simulink model "MainSim"  (R2024a)
settings: Solver=ode4  StartTime=0.0  StopTime=simtime  FixedStep=0.1  RelTol=1e-3
values from neighbouring files (symbols this model uses):
  C = [1 0 0 0 0 0 -1 0 0 0 0 0 ... (45 elements, 5x9)]    [C.mat]
undefined symbols (not defined in the file or in its folder): Ki, Kp, ssest, syys, utrim, xtrim
libraries: neural x680
(part 1 of 12)
settings Model: Creator=soeta  LastModifiedBy=soeta
settings DataIOCC: ReturnWorkspaceOutputs=off

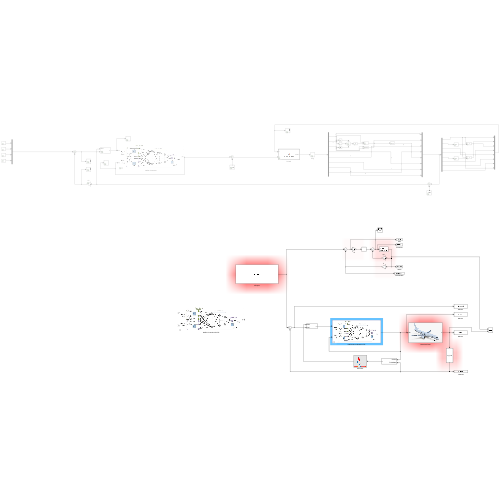
[thumbnail: Simulink's stored preview of the top-level diagram]
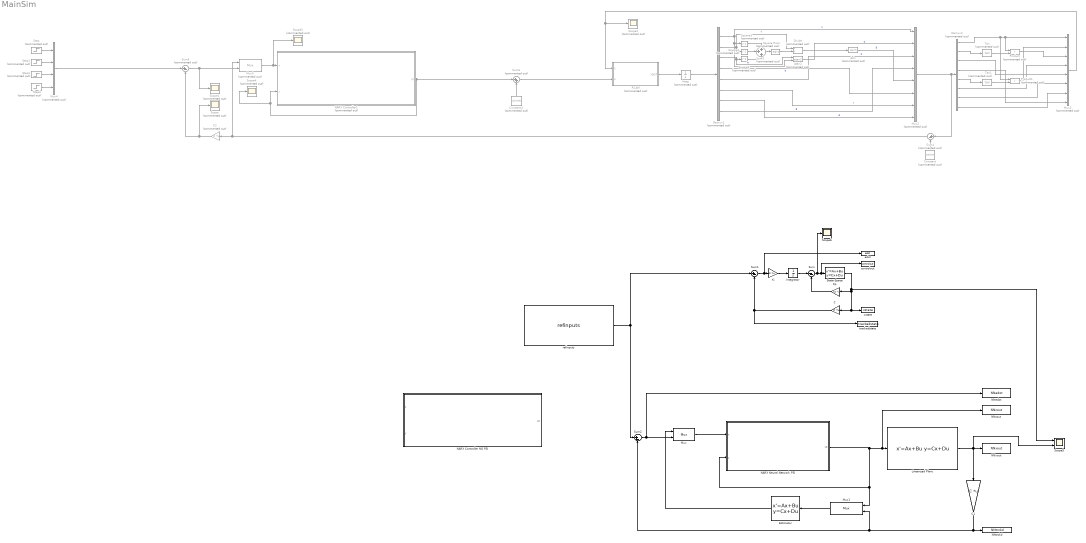
== system MainSim ==
  Asin : Trigonometry  Commented=on  Operator=asin
  Atan2 : Trigonometry  Commented=on  Operator=atan2
  C : Gain  Gain=C  Multiplication=Matrix(K*u)
  C1 : Gain  Gain=C  Multiplication=Matrix(K*u)
      mask Display: fprintf('u γ β Φ')
  C2 : Gain  Commented=on  Gain=C  Multiplication=Matrix(K*u)
  Constant : Constant  Commented=on  Value=xtrim
  Constant1 : Constant  Commented=on  Value=utrim
  Demux1 : Demux  Commented=on  Outputs=8
  Demux2 : Demux  Commented=on  Outputs=8
  Divide : Product  Commented=on  Inputs=*/
  Estimator : StateSpace  A=ssest.A  B=ssest.B  C=ssest.C  D=ssest.D  InitialCondition=0
      mask Display: image('icon_Est.png');
  Integ : Integrator  Commented=on  InitialCondition=xtrim
  Integrator : Integrator
  Ki : Gain  Gain=Ki  Multiplication=Matrix(K*u)
  Kp : Gain  Gain=Kp  Multiplication=Matrix(K*u)
  Linearized Plant : StateSpace  A=syys.A  B=syys.B  C=syys.C  D=syys.D  InitialCondition=0
      mask Display:
      | image('icon_757.png');
      | port_label('input', 1, 'δu');
      | port_label('output', 1, 'x');
  Mux : Mux  Inputs=2
      mask Display:
      | port_label('input', 1, 'Estx');
      | port_label('input', 2, 'Ref');
      | port_label('output', 1, 'x');
  Mux1 : Mux  Inputs=2
      mask Display:
      | port_label('output', 1, 'x');
      | port_label('input', 1, 'CtrlOut');
      | port_label('input', 2, 'TrckdState');
  Mux2 : Mux  Commented=on  Inputs=8
  Mux3 : Mux  Commented=on  Inputs=8
  Mux4 : Mux  Commented=on
  Mux5 : Mux  Commented=on  Inputs=2
      mask Display:
      | port_label('input', 1, 'Estx');
      | port_label('input', 2, 'Ref');
      | port_label('output', 1, 'x');
  NARX Controller NO PSI : Subsystem  mask{pi_input_1_delayed_1=[0;0;0;0;0;0;0;0;0;0;0;0], pi_input_2_delayed_1=[0;0;0;0;0]}
      mask prompts: pi_input_1_delayed_1 "Preprocessed initial input 1 state at timestep 0."; pi_input_2_delayed_1 "Preprocessed initial input 2 state at timestep 0."
      mask help: NARX Neural Network
      mask Display: image('icon_NARX.png');
  NARX Controller1 : Subsystem  Commented=on  mask{pi_input_1_delayed_1=[0;0;0;0;0;0;0;0;0;0;0;0], pi_input_2_delayed_1=[0;0;0;0;0]}
      mask prompts: pi_input_1_delayed_1 "Preprocessed initial input 1 state at timestep 0."; pi_input_2_delayed_1 "Preprocessed initial input 2 state at timestep 0."
      mask help: NARX Neural Network
      mask Display: image('icon_NARX.png');
  NARX Neural Network PSI : Subsystem  mask{pi_input_1_delayed_1=[0;0;0;0;0;0;0;0;0;0;0;0;0;0], pi_input_2_delayed_1=[0;0;0;0;0]}
      mask prompts: pi_input_1_delayed_1 "Preprocessed initial input 1 state at timestep 0."; pi_input_2_delayed_1 "Preprocessed initial input 2 state at timestep 0."
      mask help: NARX Neural Network
      mask Display:
      | e = 0.06;c1 = [120 150 230]/255;c2 = ([120 150 230]+0)/383;c3 = ([120 150 230]+128)/383;patch([0 1 1 0],[0 0 1 1],c1);patch([0 1 1 1-e 1-e 0+e],[0 0 1 1-e 0+e 0+e],c2);patch([0 0 1 1-e 0+e 0+e],[0 1 1 1-e 1-e 0+e],c3);plot([0 1 1 0 0],[0 0 1 1 0]);fprintf('NNET');port_label('input',1,' x');port_label('input',2,' y');port_label('output',1,'y2 ');
      | image('icon_NARX.png');
  NNcout : ToWorkspace  VariableName=NNcout  SaveFormat=Timeseries  SampleTime=-1
  NNedot : ToWorkspace  VariableName=NNedot  SaveFormat=Timeseries  SampleTime=-1
  NNtrckd : ToWorkspace  VariableName=NNtrckd  SaveFormat=Timeseries  SampleTime=-1
  NNxout : ToWorkspace  VariableName=NNxout  SaveFormat=Timeseries  SampleTime=-1
  Product : Product  Commented=on
  Product1 : Product  Commented=on
  RCAM : MATLAB Function  Commented=on  TreatAsAtomicUnit=on
  Scope{,1..4} (5 alike) : Scope  Commented=on
  Scope5 : Scope  NumInputPorts=2
  Scope6 : Scope
  Square Root : Sqrt  Commented=on
  Square1 : Math  Commented=on  Operator=square
  Square2 : Math  Commented=on  Operator=square
  Square3 : Math  Commented=on  Operator=square
  State-Space : StateSpace  A=syys.A  B=syys.B  C=syys.C  D=syys.D  InitialCondition=0
  Step{,1..3} (4 alike) : Step  Commented=on  Time=0  After=0  SampleTime=0
  Sum : Sum  Inputs=|--
  Sum1 : Sum  Inputs=|+-
  Sum2 : Sum  Inputs=|+-
  Sum3 : Sum  Commented=on  Inputs=+++
  Sum4 : Sum  Commented=on  Inputs=|+-
  Sum5 : Sum  Commented=on  Inputs=|+-
  Sum6 : Sum  Commented=on  Inputs=|++
  Tan : Trigonometry  Commented=on  Operator=tan
  Tan1 : Trigonometry  Commented=on  Operator=tan
  controlout : ToWorkspace  VariableName=controlout  SaveFormat=Timeseries  SampleTime=-1
  edot : ToWorkspace  VariableName=edot  SaveFormat=Timeseries  SampleTime=-1
  refinputs : FromWorkspace  VariableName=refinputs
  trackedstate : ToWorkspace  VariableName=trackedstate  SaveFormat=Timeseries  SampleTime=-1
  xstate : ToWorkspace  VariableName=xstate  SaveFormat=Timeseries  SampleTime=-1
  wires:
  Sum/1 -> Scope6/1, controlout/1, State-Space/1
  State-Space/1 -> Scope5/1, xstate/1, C/1, Kp/1
  Kp/1 -> Sum/2
  Ki/1 -> Integrator/1
  Integrator/1 -> Sum/1
  Sum1/1 -> edot/1, Ki/1
  C/1 -> trackedstate/1, Sum1/2
  refinputs/1 -> Sum2/1, Sum1/1
  NARX Neural Network PSI/1(y2) -> NARX Neural Network PSI/2(y), Mux1/1, NNcout/1, Linearized Plant/1
  Linearized Plant/1 -> C1/1, NNxout/1, Scope5/2
  Mux/1 -> NARX Neural Network PSI/1(x)
  Sum2/1 -> NNedot/1, Mux/2
  C1/1 -> Mux1/2, Sum2/2, NNtrckd/1
  Mux1/1 -> Estimator/1
  Estimator/1 -> Mux/1
  Integ/1 -> Demux1/1
  Asin/1 -> Mux2/5  "β"
  Demux1/5 -> Mux2/3  "q"
  Demux1/1 -> Square3/1, Atan2/2, Mux2/1  "u"
  Demux1/6 -> Mux2/7  "r"
  Square2/1 -> Sum3/3
  Square3/1 -> Sum3/1
  Demux1/8 -> Mux2/4  "θ"
  Sum3/1 -> Square Root/1
  Square Root/1 -> Divide/2
  Demux1/3 -> Atan2/1, Square2/1  "w"
  RCAM/1(XDOT) -> Integ/1
  Atan2/1 -> Mux2/2  "α"
  Demux1/2 -> Square1/1, Divide/1  "v"
  Demux1/4 -> Mux2/6  "p"
  Divide/1 -> Asin/1
  Mux3/1 -> RCAM/1(X), Scope2/1
  Demux1/7 -> Mux2/8  "Φ"
  Square1/1 -> Sum3/2
  Demux2/2 -> Tan/1
  Demux2/3 -> Mux3/5
  Product/1 -> Mux3/3
  Tan/1 -> Product/2
  Demux2/1 -> Product/1, Mux3/1, Product1/1
  Demux2/6 -> Mux3/4
  Demux2/7 -> Mux3/6
  Demux2/8 -> Mux3/7
  Product1/1 -> Mux3/2
  Tan1/1 -> Product1/2
  Demux2/4 -> Mux3/8
  Demux2/5 -> Tan1/1
  Constant/1 -> Sum4/2
  Mux2/1 -> Demux2/1, Sum4/1
  Sum4/1 -> Mux5/1, C2/1
  C2/1 -> Scope/1, Sum5/2
  Mux4/1 -> Sum5/1
  Step/1 -> Mux4/1
  Step1/1 -> Mux4/2
  Step2/1 -> Mux4/3
  Step3/1 -> Mux4/4
  NARX Controller1/1(y2) -> NARX Controller1/2(y), Scope4/1, Sum6/1
  Mux5/1 -> Scope3/1, NARX Controller1/1(x)
  Sum5/1 -> Scope1/1, Mux5/2
  Sum6/1 -> RCAM/2(U)
  Constant1/1 -> Sum6/2

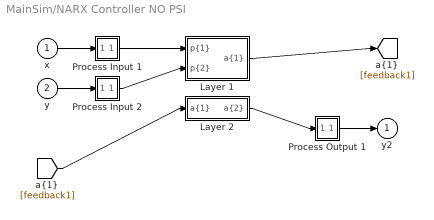
== system MainSim/NARX Controller NO PSI ==
  x : Inport  PortDimensions=12  SampleTime=0.1
      mask Display: e = 0.06;c1 = [120 230 180]/255;c2 = ([120 230 180]+0)/(256+128);c3 = ([120 230 180]+128)/(256+128);patch([0 1 1 0],[0 0 1 1],c1);patch([0 1 1 1-e 1-e 0+e],[0 0 1 1-e 0+e 0+e],c2);patch([0 0 1 1-e 0+e 0+e],[0 1 1 1-e 1-e 0+e],c3);plot([0 1 1 0 0],[0 0 1 1 0]);
  y : Inport  Port=2  PortDimensions=5  SampleTime=0.1
      mask Display: e = 0.06;c1 = [120 230 180]/255;c2 = ([120 230 180]+0)/(256+128);c3 = ([120 230 180]+128)/(256+128);patch([0 1 1 0],[0 0 1 1],c1);patch([0 1 1 1-e 1-e 0+e],[0 0 1 1-e 0+e 0+e],c2);patch([0 0 1 1-e 0+e 0+e],[0 1 1 1-e 1-e 0+e],c3);plot([0 1 1 0 0],[0 0 1 1 0]);
  Layer 1 : Subsystem
      mask Display: e = 0.06;c1 = [120 150 230]/255;c2 = ([120 150 230]+0)/383;c3 = ([120 150 230]+128)/383;patch([0 1 1 0],[0 0 1 1],c1);patch([0 1 1 1-e 1-e 0+e],[0 0 1 1-e 0+e 0+e],c2);patch([0 0 1 1-e 0+e 0+e],[0 1 1 1-e 1-e 0+e],c3);plot([0 1 1 0 0],[0 0 1 1 0]);
  Layer 2 : Subsystem
      mask Display: e = 0.06;c1 = [120 150 230]/255;c2 = ([120 150 230]+0)/383;c3 = ([120 150 230]+128)/383;patch([0 1 1 0],[0 0 1 1],c1);patch([0 1 1 1-e 1-e 0+e],[0 0 1 1-e 0+e 0+e],c2);patch([0 0 1 1-e 0+e 0+e],[0 1 1 1-e 1-e 0+e],c3);plot([0 1 1 0 0],[0 0 1 1 0]);
  Process Input 1 : Subsystem
      mask Display: e = 0.06;c1 = [120 150 230]/255;c2 = ([120 150 230]+0)/383;c3 = ([120 150 230]+128)/383;patch([0 1 1 0],[0 0 1 1],c1);patch([0 1 1 1-e 1-e 0+e],[0 0 1 1-e 0+e 0+e],c2);patch([0 0 1 1-e 0+e 0+e],[0 1 1 1-e 1-e 0+e],c3);plot([0 1 1 0 0],[0 0 1 1 0]);
  Process Input 2 : Subsystem
      mask Display: e = 0.06;c1 = [120 150 230]/255;c2 = ([120 150 230]+0)/383;c3 = ([120 150 230]+128)/383;patch([0 1 1 0],[0 0 1 1],c1);patch([0 1 1 1-e 1-e 0+e],[0 0 1 1-e 0+e 0+e],c2);patch([0 0 1 1-e 0+e 0+e],[0 1 1 1-e 1-e 0+e],c3);plot([0 1 1 0 0],[0 0 1 1 0]);
  Process Output 1 : Subsystem
      mask Display: e = 0.06;c1 = [120 150 230]/255;c2 = ([120 150 230]+0)/383;c3 = ([120 150 230]+128)/383;patch([0 1 1 0],[0 0 1 1],c1);patch([0 1 1 1-e 1-e 0+e],[0 0 1 1-e 0+e 0+e],c2);patch([0 0 1 1-e 0+e 0+e],[0 1 1 1-e 1-e 0+e],c3);plot([0 1 1 0 0],[0 0 1 1 0]);
  y2 : Outport  InitialOutput=[0;0;0;0;0]
      mask Display: e = 0.06;c1 = [120 230 180]/255;c2 = ([120 230 180]+0)/(256+128);c3 = ([120 230 180]+128)/(256+128);patch([0 1 1 0],[0 0 1 1],c1);patch([0 1 1 1-e 1-e 0+e],[0 0 1 1-e 0+e 0+e],c2);patch([0 0 1 1-e 0+e 0+e],[0 1 1 1-e 1-e 0+e],c3);plot([0 1 1 0 0],[0 0 1 1 0]);
  wires:
  Layer 2/1("a{2}") -> Process Output 1/1(a)
  [feedback1] -> Layer 2/1("a{1} ")
  Layer 1/1("a{1}") -> [feedback1]
  Process Input 2/1(p) -> Layer 1/2("p{2}")
  Process Input 1/1(p) -> Layer 1/1("p{1}")
  Process Output 1/1(y) -> y2/1
  y/1 -> Process Input 2/1(x)
  x/1 -> Process Input 1/1(x)

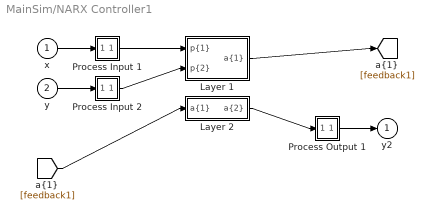
== system MainSim/NARX Controller1 ==
  x : Inport  PortDimensions=12  SampleTime=0.1
      mask Display: e = 0.06;c1 = [120 230 180]/255;c2 = ([120 230 180]+0)/(256+128);c3 = ([120 230 180]+128)/(256+128);patch([0 1 1 0],[0 0 1 1],c1);patch([0 1 1 1-e 1-e 0+e],[0 0 1 1-e 0+e 0+e],c2);patch([0 0 1 1-e 0+e 0+e],[0 1 1 1-e 1-e 0+e],c3);plot([0 1 1 0 0],[0 0 1 1 0]);
  y : Inport  Port=2  PortDimensions=5  SampleTime=0.1
      mask Display: e = 0.06;c1 = [120 230 180]/255;c2 = ([120 230 180]+0)/(256+128);c3 = ([120 230 180]+128)/(256+128);patch([0 1 1 0],[0 0 1 1],c1);patch([0 1 1 1-e 1-e 0+e],[0 0 1 1-e 0+e 0+e],c2);patch([0 0 1 1-e 0+e 0+e],[0 1 1 1-e 1-e 0+e],c3);plot([0 1 1 0 0],[0 0 1 1 0]);
  Layer 1 : Subsystem
      mask Display: e = 0.06;c1 = [120 150 230]/255;c2 = ([120 150 230]+0)/383;c3 = ([120 150 230]+128)/383;patch([0 1 1 0],[0 0 1 1],c1);patch([0 1 1 1-e 1-e 0+e],[0 0 1 1-e 0+e 0+e],c2);patch([0 0 1 1-e 0+e 0+e],[0 1 1 1-e 1-e 0+e],c3);plot([0 1 1 0 0],[0 0 1 1 0]);
  Layer 2 : Subsystem
      mask Display: e = 0.06;c1 = [120 150 230]/255;c2 = ([120 150 230]+0)/383;c3 = ([120 150 230]+128)/383;patch([0 1 1 0],[0 0 1 1],c1);patch([0 1 1 1-e 1-e 0+e],[0 0 1 1-e 0+e 0+e],c2);patch([0 0 1 1-e 0+e 0+e],[0 1 1 1-e 1-e 0+e],c3);plot([0 1 1 0 0],[0 0 1 1 0]);
  Process Input 1 : Subsystem
      mask Display: e = 0.06;c1 = [120 150 230]/255;c2 = ([120 150 230]+0)/383;c3 = ([120 150 230]+128)/383;patch([0 1 1 0],[0 0 1 1],c1);patch([0 1 1 1-e 1-e 0+e],[0 0 1 1-e 0+e 0+e],c2);patch([0 0 1 1-e 0+e 0+e],[0 1 1 1-e 1-e 0+e],c3);plot([0 1 1 0 0],[0 0 1 1 0]);
  Process Input 2 : Subsystem
      mask Display: e = 0.06;c1 = [120 150 230]/255;c2 = ([120 150 230]+0)/383;c3 = ([120 150 230]+128)/383;patch([0 1 1 0],[0 0 1 1],c1);patch([0 1 1 1-e 1-e 0+e],[0 0 1 1-e 0+e 0+e],c2);patch([0 0 1 1-e 0+e 0+e],[0 1 1 1-e 1-e 0+e],c3);plot([0 1 1 0 0],[0 0 1 1 0]);
  Process Output 1 : Subsystem
      mask Display: e = 0.06;c1 = [120 150 230]/255;c2 = ([120 150 230]+0)/383;c3 = ([120 150 230]+128)/383;patch([0 1 1 0],[0 0 1 1],c1);patch([0 1 1 1-e 1-e 0+e],[0 0 1 1-e 0+e 0+e],c2);patch([0 0 1 1-e 0+e 0+e],[0 1 1 1-e 1-e 0+e],c3);plot([0 1 1 0 0],[0 0 1 1 0]);
  y2 : Outport  InitialOutput=[0;0;0;0;0]
      mask Display: e = 0.06;c1 = [120 230 180]/255;c2 = ([120 230 180]+0)/(256+128);c3 = ([120 230 180]+128)/(256+128);patch([0 1 1 0],[0 0 1 1],c1);patch([0 1 1 1-e 1-e 0+e],[0 0 1 1-e 0+e 0+e],c2);patch([0 0 1 1-e 0+e 0+e],[0 1 1 1-e 1-e 0+e],c3);plot([0 1 1 0 0],[0 0 1 1 0]);
  wires:
  Layer 2/1("a{2}") -> Process Output 1/1(a)
  [feedback1] -> Layer 2/1("a{1} ")
  Layer 1/1("a{1}") -> [feedback1]
  Process Input 2/1(p) -> Layer 1/2("p{2}")
  Process Input 1/1(p) -> Layer 1/1("p{1}")
  Process Output 1/1(y) -> y2/1
  y/1 -> Process Input 2/1(x)
  x/1 -> Process Input 1/1(x)

== system MainSim/NARX Neural Network PSI ==
  x : Inport  PortDimensions=14  SampleTime=0.1
      mask Display: e = 0.06;c1 = [120 230 180]/255;c2 = ([120 230 180]+0)/(256+128);c3 = ([120 230 180]+128)/(256+128);patch([0 1 1 0],[0 0 1 1],c1);patch([0 1 1 1-e 1-e 0+e],[0 0 1 1-e 0+e 0+e],c2);patch([0 0 1 1-e 0+e 0+e],[0 1 1 1-e 1-e 0+e],c3);plot([0 1 1 0 0],[0 0 1 1 0]);
  y : Inport  Port=2  PortDimensions=5  SampleTime=0.1
      mask Display: e = 0.06;c1 = [120 230 180]/255;c2 = ([120 230 180]+0)/(256+128);c3 = ([120 230 180]+128)/(256+128);patch([0 1 1 0],[0 0 1 1],c1);patch([0 1 1 1-e 1-e 0+e],[0 0 1 1-e 0+e 0+e],c2);patch([0 0 1 1-e 0+e 0+e],[0 1 1 1-e 1-e 0+e],c3);plot([0 1 1 0 0],[0 0 1 1 0]);
  Layer 1 : Subsystem
      mask Display: e = 0.06;c1 = [120 150 230]/255;c2 = ([120 150 230]+0)/383;c3 = ([120 150 230]+128)/383;patch([0 1 1 0],[0 0 1 1],c1);patch([0 1 1 1-e 1-e 0+e],[0 0 1 1-e 0+e 0+e],c2);patch([0 0 1 1-e 0+e 0+e],[0 1 1 1-e 1-e 0+e],c3);plot([0 1 1 0 0],[0 0 1 1 0]);
  Layer 2 : Subsystem
      mask Display: e = 0.06;c1 = [120 150 230]/255;c2 = ([120 150 230]+0)/383;c3 = ([120 150 230]+128)/383;patch([0 1 1 0],[0 0 1 1],c1);patch([0 1 1 1-e 1-e 0+e],[0 0 1 1-e 0+e 0+e],c2);patch([0 0 1 1-e 0+e 0+e],[0 1 1 1-e 1-e 0+e],c3);plot([0 1 1 0 0],[0 0 1 1 0]);
  Process Input 1 : Subsystem
      mask Display: e = 0.06;c1 = [120 150 230]/255;c2 = ([120 150 230]+0)/383;c3 = ([120 150 230]+128)/383;patch([0 1 1 0],[0 0 1 1],c1);patch([0 1 1 1-e 1-e 0+e],[0 0 1 1-e 0+e 0+e],c2);patch([0 0 1 1-e 0+e 0+e],[0 1 1 1-e 1-e 0+e],c3);plot([0 1 1 0 0],[0 0 1 1 0]);
  Process Input 2 : Subsystem
      mask Display: e = 0.06;c1 = [120 150 230]/255;c2 = ([120 150 230]+0)/383;c3 = ([120 150 230]+128)/383;patch([0 1 1 0],[0 0 1 1],c1);patch([0 1 1 1-e 1-e 0+e],[0 0 1 1-e 0+e 0+e],c2);patch([0 0 1 1-e 0+e 0+e],[0 1 1 1-e 1-e 0+e],c3);plot([0 1 1 0 0],[0 0 1 1 0]);
  Process Output 1 : Subsystem
      mask Display: e = 0.06;c1 = [120 150 230]/255;c2 = ([120 150 230]+0)/383;c3 = ([120 150 230]+128)/383;patch([0 1 1 0],[0 0 1 1],c1);patch([0 1 1 1-e 1-e 0+e],[0 0 1 1-e 0+e 0+e],c2);patch([0 0 1 1-e 0+e 0+e],[0 1 1 1-e 1-e 0+e],c3);plot([0 1 1 0 0],[0 0 1 1 0]);
  y2 : Outport  InitialOutput=[0;0;0;0;0]
      mask Display: e = 0.06;c1 = [120 230 180]/255;c2 = ([120 230 180]+0)/(256+128);c3 = ([120 230 180]+128)/(256+128);patch([0 1 1 0],[0 0 1 1],c1);patch([0 1 1 1-e 1-e 0+e],[0 0 1 1-e 0+e 0+e],c2);patch([0 0 1 1-e 0+e 0+e],[0 1 1 1-e 1-e 0+e],c3);plot([0 1 1 0 0],[0 0 1 1 0]);
  wires:
  Layer 2/1("a{2}") -> Process Output 1/1(a)
  [feedback1] -> Layer 2/1("a{1} ")
  Layer 1/1("a{1}") -> [feedback1]
  Process Input 2/1(p) -> Layer 1/2("p{2}")
  Process Input 1/1(p) -> Layer 1/1("p{1}")
  Process Output 1/1(y) -> y2/1
  y/1 -> Process Input 2/1(x)
  x/1 -> Process Input 1/1(x)

== system MainSim/NARX Controller NO PSI/Layer 1 ==
  "p{1}" : Inport  PortDimensions=12  SampleTime=0.1
      mask Display: e = 0.06;c1 = [120 230 180]/255;c2 = ([120 230 180]+0)/(256+128);c3 = ([120 230 180]+128)/(256+128);patch([0 1 1 0],[0 0 1 1],c1);patch([0 1 1 1-e 1-e 0+e],[0 0 1 1-e 0+e 0+e],c2);patch([0 0 1 1-e 0+e 0+e],[0 1 1 1-e 1-e 0+e],c3);plot([0 1 1 0 0],[0 0 1 1 0]);
  "p{2}" : Inport  Port=2  PortDimensions=5  SampleTime=0.1
      mask Display: e = 0.06;c1 = [120 230 180]/255;c2 = ([120 230 180]+0)/(256+128);c3 = ([120 230 180]+128)/(256+128);patch([0 1 1 0],[0 0 1 1],c1);patch([0 1 1 1-e 1-e 0+e],[0 0 1 1-e 0+e 0+e],c2);patch([0 0 1 1-e 0+e 0+e],[0 1 1 1-e 1-e 0+e],c3);plot([0 1 1 0 0],[0 0 1 1 0]);
  Delays 1 : Subsystem
      mask Display: e = 0.06;c1 = [120 150 230]/255;c2 = ([120 150 230]+0)/383;c3 = ([120 150 230]+128)/383;patch([0 1 1 0],[0 0 1 1],c1);patch([0 1 1 1-e 1-e 0+e],[0 0 1 1-e 0+e 0+e],c2);patch([0 0 1 1-e 0+e 0+e],[0 1 1 1-e 1-e 0+e],c3);plot([0 1 1 0 0],[0 0 1 1 0]);disp('1');
  Delays 2 : Subsystem
      mask Display: e = 0.06;c1 = [120 150 230]/255;c2 = ([120 150 230]+0)/383;c3 = ([120 150 230]+128)/383;patch([0 1 1 0],[0 0 1 1],c1);patch([0 1 1 1-e 1-e 0+e],[0 0 1 1-e 0+e 0+e],c2);patch([0 0 1 1-e 0+e 0+e],[0 1 1 1-e 1-e 0+e],c3);plot([0 1 1 0 0],[0 0 1 1 0]);disp('1');
  "IW{1,1}" : Subsystem
      mask Display: e = 0.06;c1 = [120 150 230]/255;c2 = ([120 150 230]+0)/383;c3 = ([120 150 230]+128)/383;patch([0 1 1 0],[0 0 1 1],c1);patch([0 1 1 1-e 1-e 0+e],[0 0 1 1-e 0+e 0+e],c2);patch([0 0 1 1-e 0+e 0+e],[0 1 1 1-e 1-e 0+e],c3);plot([0 1 1 0 0],[0 0 1 1 0]);disp('W');
  "IW{1,2}" : Subsystem
      mask Display: e = 0.06;c1 = [120 150 230]/255;c2 = ([120 150 230]+0)/383;c3 = ([120 150 230]+128)/383;patch([0 1 1 0],[0 0 1 1],c1);patch([0 1 1 1-e 1-e 0+e],[0 0 1 1-e 0+e 0+e],c2);patch([0 0 1 1-e 0+e 0+e],[0 1 1 1-e 1-e 0+e],c3);plot([0 1 1 0 0],[0 0 1 1 0]);disp('W');
  "b{1}" : Constant  Value=[-0.007554334213848506833499651946794983814470469951629638671875;-0.01028875835034793496947091995252776541747152805328369140625;-0.006755015401667272857688661957809017621912062168121337890625;-0.00819595428001762722758360979469216545112431049346923828125;-0.0012098008006652060351837629781357463798485696315765380859375;0.0114355734405583477075740717054941342212259769439697265625;-0.00825606250588458399908287077550994581542909145355224609375;0.00960914980064617695043605039018075331114232540130615234375;0.01665836603007038452251009630344924516975879669189453125;-0.01245531687480195930095572265372538822703063488006591796875;0.01205156321038763043984598510860450915060937404632568359375;0.01278715178153389496473746334004317759536206722259521484375;0.01115871878165029806861952010876848362386226654052734375;-0.002859971099156568587196236563841011957265436649322509765625;-0.0019629482754365619630310124676952909794636070728302001953125;-0.0086151839933822187134193626434353063814342021942138671875;0.00174858440777187038213391634400295515661127865314483642578125;-0.01323180367395891676718377993893227539956569671630859375;0.00276938240801051678563471369898252305574715137481689453125;-0.00877533941830567661146478286582350847311317920684814453125;0.00268341621277570600845319148675116593949496746063232421875;0.0078330097519283721496652361793167074210941791534423828125;0.01056608133068198847326346623276549507863819599151611328125;0.00856310439247244363503153152805680292658507823944091796875;0.0037300890089778195903014168521849569515325129032135009765625;-0.0036564673780585909938778410577242539147846400737762451171875;0.00910931066802874063459416476007390883751213550567626953125;-0.004678353366452448793000318261192660429514944553375244140625;-0.0080094426535534286870632314503382076509296894073486328125;-0.0007558791140228862844019364075620615039952099323272705078125;0.006449121773167149594685465530119472532533109188079833984375;-0.00131600111876151756699904193936845331336371600627899169921875;0.00525732431395188604117407749072299338877201080322265625;0.001332551688508547445277674370345266652293503284454345703125;0.00427706480160073253260488712612641393207013607025146484375;-0.00950556679029437336103658395813909010030329227447509765625;0.005730426808411771821827329631560132838785648345947265625;0.00508392544602999894853834206287501729093492031097412109375;0.00506058440005886268908685821088511147536337375640869140625;0.011834339263637465300416096170010860078036785125732421875;-0.0003449992763752953383281363297641064491472207009792327880859375;-0.0114351107070735542869943657251496915705502033233642578125;0.00783101165138963377365666218565820599906146526336669921875;-0.01403100732721834949245920398652742733247578144073486328125;-0.004373402040658883570267700946487821056507527828216552734375;0.00822243007501474894305193430454892222769558429718017578125;-0.00102351186185454059475452570637798999086953699588775634765625;0.009431169907436365296149460846208967268466949462890625;0.0063451948741047557722705363403292722068727016448974609375;0.0041419120969572974233496864826520322822034358978271484375;-0.0035233659709833216149010848283751329290680587291717529296875;0.0116054220619492449995124871975349378772079944610595703125;-0.012943434681874775582510750382425612770020961761474609375;-0.01144783414304829764762683197432124870829284191131591796875;-0.0245514420394156891724879443472673301585018634796142578125;-0.005883344458003751664687541733655962161719799041748046875;0.00166971111128907793476339183058598791831173002719879150390625;0.0122237284889527286768640124137164093554019927978515625;0.01372193035965791653441048225658960291184484958648681640625;-0.006650703206520082282071637536091657239012420177459716796875;-0.00979041929095626935197760332130201277323067188262939453125;0.0018736226966915531071122824613439661334268748760223388671875;0.009417437572067553774868287064236938022077083587646484375;-0.01170226028499656012460405918318429030478000640869140625 ...(+2243 chars)]
      mask Display: e = 0.06;c1 = [120 150 230]/255;c2 = ([120 150 230]+0)/383;c3 = ([120 150 230]+128)/383;patch([0 1 1 0],[0 0 1 1],c1);patch([0 1 1 1-e 1-e 0+e],[0 0 1 1-e 0+e 0+e],c2);patch([0 0 1 1-e 0+e 0+e],[0 1 1 1-e 1-e 0+e],c3);plot([0 1 1 0 0],[0 0 1 1 0]);disp('b');
  netsum : Sum  Inputs=3  InputSameDT=on  SaturateOnIntegerOverflow=on  OutDataTypeStr=Inherit: Same as first input
      mask Display: e = 0.06;c1 = [120 150 230]/255;c2 = ([120 150 230]+0)/383;c3 = ([120 150 230]+128)/383;patch([0 1 1 0],[0 0 1 1],c1);patch([0 1 1 1-e 1-e 0+e],[0 0 1 1-e 0+e 0+e],c2);patch([0 0 1 1-e 0+e 0+e],[0 1 1 1-e 1-e 0+e],c3);plot([0 1 1 0 0],[0 0 1 1 0]);disp('+');
  tansig : neural/Transfer Functions/tansig
  "a{1}" : Outport  InitialOutput=[0;0;0;0;0;0;0;0;0;0;0;0;0;0;0;0;0;0;0;0;0;0;0;0;0;0;0;0;0;0;0;0;0;0;0;0;0;0;0;0;0;0;0;0;0;0;0;0;0;0;0;0;0;0;0;0;0;0;0;0;0;0;0;0;0;0;0;0;0;0;0;0;0;0;0;0;0;0;0;0;0;0;0;0;0;0;0;0;0;0;0;0;0;0;0;0;0;0;0;0]
      mask Display: e = 0.06;c1 = [120 230 180]/255;c2 = ([120 230 180]+0)/(256+128);c3 = ([120 230 180]+128)/(256+128);patch([0 1 1 0],[0 0 1 1],c1);patch([0 1 1 1-e 1-e 0+e],[0 0 1 1-e 0+e 0+e],c2);patch([0 0 1 1-e 0+e 0+e],[0 1 1 1-e 1-e 0+e],c3);plot([0 1 1 0 0],[0 0 1 1 0]);
  wires:
  tansig/1 -> "a{1}"/1
  netsum/1 -> tansig/1
  "b{1}"/1 -> netsum/3
  "IW{1,2}"/1("iz{1,2}") -> netsum/2
  Delays 2/1("pd{1,2}") -> "IW{1,2}"/1("pd{1,2}")
  "p{2}"/1 -> Delays 2/1("p{1}")
  "IW{1,1}"/1("iz{1,1}") -> netsum/1
  Delays 1/1("pd{1,1}") -> "IW{1,1}"/1("pd{1,1}")
  "p{1}"/1 -> Delays 1/1("p{1}")

== system MainSim/NARX Controller NO PSI/Layer 2 ==
  "a{1} " : Inport  PortDimensions=100  SampleTime=0.1
      mask Display: e = 0.06;c1 = [120 230 180]/255;c2 = ([120 230 180]+0)/(256+128);c3 = ([120 230 180]+128)/(256+128);patch([0 1 1 0],[0 0 1 1],c1);patch([0 1 1 1-e 1-e 0+e],[0 0 1 1-e 0+e 0+e],c2);patch([0 0 1 1-e 0+e 0+e],[0 1 1 1-e 1-e 0+e],c3);plot([0 1 1 0 0],[0 0 1 1 0]);
  Delays 1 : Subsystem
      mask Display: e = 0.06;c1 = [120 150 230]/255;c2 = ([120 150 230]+0)/383;c3 = ([120 150 230]+128)/383;patch([0 1 1 0],[0 0 1 1],c1);patch([0 1 1 1-e 1-e 0+e],[0 0 1 1-e 0+e 0+e],c2);patch([0 0 1 1-e 0+e 0+e],[0 1 1 1-e 1-e 0+e],c3);plot([0 1 1 0 0],[0 0 1 1 0]);disp('0');
  "LW{2,1}" : Subsystem
      mask Display: e = 0.06;c1 = [120 150 230]/255;c2 = ([120 150 230]+0)/383;c3 = ([120 150 230]+128)/383;patch([0 1 1 0],[0 0 1 1],c1);patch([0 1 1 1-e 1-e 0+e],[0 0 1 1-e 0+e 0+e],c2);patch([0 0 1 1-e 0+e 0+e],[0 1 1 1-e 1-e 0+e],c3);plot([0 1 1 0 0],[0 0 1 1 0]);disp('W');
  "b{2}" : Constant  Value=[-0.038746412276604295932269650393209303729236125946044921875;0.10887518811133491125620054162936867214739322662353515625;-0.04051718221217563697944541445394861511886119842529296875;-0.041253916418590740045058140594846918247640132904052734375;0.041980855311955021791359143890076666139066219329833984375]
      mask Display: e = 0.06;c1 = [120 150 230]/255;c2 = ([120 150 230]+0)/383;c3 = ([120 150 230]+128)/383;patch([0 1 1 0],[0 0 1 1],c1);patch([0 1 1 1-e 1-e 0+e],[0 0 1 1-e 0+e 0+e],c2);patch([0 0 1 1-e 0+e 0+e],[0 1 1 1-e 1-e 0+e],c3);plot([0 1 1 0 0],[0 0 1 1 0]);disp('b');
  netsum : Sum  Inputs=2  InputSameDT=on  SaturateOnIntegerOverflow=on  OutDataTypeStr=Inherit: Same as first input
      mask Display: e = 0.06;c1 = [120 150 230]/255;c2 = ([120 150 230]+0)/383;c3 = ([120 150 230]+128)/383;patch([0 1 1 0],[0 0 1 1],c1);patch([0 1 1 1-e 1-e 0+e],[0 0 1 1-e 0+e 0+e],c2);patch([0 0 1 1-e 0+e 0+e],[0 1 1 1-e 1-e 0+e],c3);plot([0 1 1 0 0],[0 0 1 1 0]);disp('+');
  purelin : neural/Transfer Functions/purelin
  "a{2}" : Outport  InitialOutput=[0;0;0;0;0]
      mask Display: e = 0.06;c1 = [120 230 180]/255;c2 = ([120 230 180]+0)/(256+128);c3 = ([120 230 180]+128)/(256+128);patch([0 1 1 0],[0 0 1 1],c1);patch([0 1 1 1-e 1-e 0+e],[0 0 1 1-e 0+e 0+e],c2);patch([0 0 1 1-e 0+e 0+e],[0 1 1 1-e 1-e 0+e],c3);plot([0 1 1 0 0],[0 0 1 1 0]);
  wires:
  purelin/1 -> "a{2}"/1
  netsum/1 -> purelin/1
  "b{2}"/1 -> netsum/2
  "LW{2,1}"/1("lz{2,1}") -> netsum/1
  Delays 1/1("pd{2,1}") -> "LW{2,1}"/1("ad{2,1}")
  "a{1} "/1 -> Delays 1/1("p{2}")

== system MainSim/NARX Controller NO PSI/Process Input 1 ==
  x : Inport  PortDimensions=12  SampleTime=0.1
      mask Display: e = 0.06;c1 = [120 230 180]/255;c2 = ([120 230 180]+0)/(256+128);c3 = ([120 230 180]+128)/(256+128);patch([0 1 1 0],[0 0 1 1],c1);patch([0 1 1 1-e 1-e 0+e],[0 0 1 1-e 0+e 0+e],c2);patch([0 0 1 1-e 0+e 0+e],[0 1 1 1-e 1-e 0+e],c3);plot([0 1 1 0 0],[0 0 1 1 0]);
  mapminmax : neural/Processing Functions/mapminmax  xmin=[-0.0129651907970248399248891502111;-0.169102256865743955094316675059;-0.000261394129407086525749420724551;-0.000200456542083920537114863358319;-0.0572538413172016327767899213086;-0.00259145694524988380244567842681;-0.00814332636769390071085350513158;-0.000996740230341396863528169447477;-0.0513394595556882285536381971269;-0.0447646016402733909478328655496;-0.052963182292912053261701998963;-0.0100089877342308310875784727045]  xmax=[0.0513394595556882285536381971269;0.00399453634531498312509878445553;6.63522293856221414068419228727e-05;0.00596627424954731047646028230247;0.0572499038085891240323910267307;0.00262231786722454379007229974263;0.000519043447362519381506340554466;0.0105862926184974084214962530837;0.0499577765287277028583012850049;0.177237932971395034664752188291;0.0529671449844292679953738911536;0.00997102928949204769804026682323]  ymin=-1  ymax=1
  p : Outport  PortDimensions=12  SampleTime=0.1
      mask Display: e = 0.06;c1 = [120 230 180]/255;c2 = ([120 230 180]+0)/(256+128);c3 = ([120 230 180]+128)/(256+128);patch([0 1 1 0],[0 0 1 1],c1);patch([0 1 1 1-e 1-e 0+e],[0 0 1 1-e 0+e 0+e],c2);patch([0 0 1 1-e 0+e 0+e],[0 1 1 1-e 1-e 0+e],c3);plot([0 1 1 0 0],[0 0 1 1 0]);
  wires:
  mapminmax/1 -> p/1
  x/1 -> mapminmax/1

== system MainSim/NARX Controller NO PSI/Process Input 2 ==
  x : Inport  PortDimensions=5  SampleTime=0.1
      mask Display: e = 0.06;c1 = [120 230 180]/255;c2 = ([120 230 180]+0)/(256+128);c3 = ([120 230 180]+128)/(256+128);patch([0 1 1 0],[0 0 1 1],c1);patch([0 1 1 1-e 1-e 0+e],[0 0 1 1-e 0+e 0+e],c2);patch([0 0 1 1-e 0+e 0+e],[0 1 1 1-e 1-e 0+e],c3);plot([0 1 1 0 0],[0 0 1 1 0]);
  mapminmax : neural/Processing Functions/mapminmax  xmin=[-0.20244393015821871006920673608;-0.000162983708575139977017820491767;-0.493690097282159567892989571192;-0.2162391512775998225759366278;-0.00605850883196610689312988640154]  xmax=[0.00478930326934306517527861757344;0.00152521114561354753647037796327;0.0115063547556192961873744451395;0.00507127823624882630160204399772;0.226011889004929134028287762703]  ymin=-1  ymax=1
  p : Outport  PortDimensions=5  SampleTime=0.1
      mask Display: e = 0.06;c1 = [120 230 180]/255;c2 = ([120 230 180]+0)/(256+128);c3 = ([120 230 180]+128)/(256+128);patch([0 1 1 0],[0 0 1 1],c1);patch([0 1 1 1-e 1-e 0+e],[0 0 1 1-e 0+e 0+e],c2);patch([0 0 1 1-e 0+e 0+e],[0 1 1 1-e 1-e 0+e],c3);plot([0 1 1 0 0],[0 0 1 1 0]);
  wires:
  mapminmax/1 -> p/1
  x/1 -> mapminmax/1

== system MainSim/NARX Controller NO PSI/Process Output 1 ==
  a : Inport  PortDimensions=5  SampleTime=0.1
      mask Display: e = 0.06;c1 = [120 230 180]/255;c2 = ([120 230 180]+0)/(256+128);c3 = ([120 230 180]+128)/(256+128);patch([0 1 1 0],[0 0 1 1],c1);patch([0 1 1 1-e 1-e 0+e],[0 0 1 1-e 0+e 0+e],c2);patch([0 0 1 1-e 0+e 0+e],[0 1 1 1-e 1-e 0+e],c3);plot([0 1 1 0 0],[0 0 1 1 0]);
  mapminmax_reverse : neural/Processing Functions/mapminmax_reverse  xmin=[-0.20244393015821871006920673608;-0.000162983708575139977017820491767;-0.493690097282159567892989571192;-0.2162391512775998225759366278;-0.00605850883196610689312988640154]  xmax=[0.00478930326934306517527861757344;0.00152521114561354753647037796327;0.0115063547556192961873744451395;0.00507127823624882630160204399772;0.226011889004929134028287762703]  ymin=-1  ymax=1
  y : Outport  PortDimensions=5  SampleTime=0.1
      mask Display: e = 0.06;c1 = [120 230 180]/255;c2 = ([120 230 180]+0)/(256+128);c3 = ([120 230 180]+128)/(256+128);patch([0 1 1 0],[0 0 1 1],c1);patch([0 1 1 1-e 1-e 0+e],[0 0 1 1-e 0+e 0+e],c2);patch([0 0 1 1-e 0+e 0+e],[0 1 1 1-e 1-e 0+e],c3);plot([0 1 1 0 0],[0 0 1 1 0]);
  wires:
  mapminmax_reverse/1 -> y/1
  a/1 -> mapminmax_reverse/1

== system MainSim/NARX Controller1/Layer 1 ==
  "p{1}" : Inport  PortDimensions=12  SampleTime=0.1
      mask Display: e = 0.06;c1 = [120 230 180]/255;c2 = ([120 230 180]+0)/(256+128);c3 = ([120 230 180]+128)/(256+128);patch([0 1 1 0],[0 0 1 1],c1);patch([0 1 1 1-e 1-e 0+e],[0 0 1 1-e 0+e 0+e],c2);patch([0 0 1 1-e 0+e 0+e],[0 1 1 1-e 1-e 0+e],c3);plot([0 1 1 0 0],[0 0 1 1 0]);
  "p{2}" : Inport  Port=2  PortDimensions=5  SampleTime=0.1
      mask Display: e = 0.06;c1 = [120 230 180]/255;c2 = ([120 230 180]+0)/(256+128);c3 = ([120 230 180]+128)/(256+128);patch([0 1 1 0],[0 0 1 1],c1);patch([0 1 1 1-e 1-e 0+e],[0 0 1 1-e 0+e 0+e],c2);patch([0 0 1 1-e 0+e 0+e],[0 1 1 1-e 1-e 0+e],c3);plot([0 1 1 0 0],[0 0 1 1 0]);
  Delays 1 : Subsystem
      mask Display: e = 0.06;c1 = [120 150 230]/255;c2 = ([120 150 230]+0)/383;c3 = ([120 150 230]+128)/383;patch([0 1 1 0],[0 0 1 1],c1);patch([0 1 1 1-e 1-e 0+e],[0 0 1 1-e 0+e 0+e],c2);patch([0 0 1 1-e 0+e 0+e],[0 1 1 1-e 1-e 0+e],c3);plot([0 1 1 0 0],[0 0 1 1 0]);disp('1');
  Delays 2 : Subsystem
      mask Display: e = 0.06;c1 = [120 150 230]/255;c2 = ([120 150 230]+0)/383;c3 = ([120 150 230]+128)/383;patch([0 1 1 0],[0 0 1 1],c1);patch([0 1 1 1-e 1-e 0+e],[0 0 1 1-e 0+e 0+e],c2);patch([0 0 1 1-e 0+e 0+e],[0 1 1 1-e 1-e 0+e],c3);plot([0 1 1 0 0],[0 0 1 1 0]);disp('1');
  "IW{1,1}" : Subsystem
      mask Display: e = 0.06;c1 = [120 150 230]/255;c2 = ([120 150 230]+0)/383;c3 = ([120 150 230]+128)/383;patch([0 1 1 0],[0 0 1 1],c1);patch([0 1 1 1-e 1-e 0+e],[0 0 1 1-e 0+e 0+e],c2);patch([0 0 1 1-e 0+e 0+e],[0 1 1 1-e 1-e 0+e],c3);plot([0 1 1 0 0],[0 0 1 1 0]);disp('W');
  "IW{1,2}" : Subsystem
      mask Display: e = 0.06;c1 = [120 150 230]/255;c2 = ([120 150 230]+0)/383;c3 = ([120 150 230]+128)/383;patch([0 1 1 0],[0 0 1 1],c1);patch([0 1 1 1-e 1-e 0+e],[0 0 1 1-e 0+e 0+e],c2);patch([0 0 1 1-e 0+e 0+e],[0 1 1 1-e 1-e 0+e],c3);plot([0 1 1 0 0],[0 0 1 1 0]);disp('W');
  "b{1}" : Constant  Value=[-0.007554334213848506833499651946794983814470469951629638671875;-0.01028875835034793496947091995252776541747152805328369140625;-0.006755015401667272857688661957809017621912062168121337890625;-0.00819595428001762722758360979469216545112431049346923828125;-0.0012098008006652060351837629781357463798485696315765380859375;0.0114355734405583477075740717054941342212259769439697265625;-0.00825606250588458399908287077550994581542909145355224609375;0.00960914980064617695043605039018075331114232540130615234375;0.01665836603007038452251009630344924516975879669189453125;-0.01245531687480195930095572265372538822703063488006591796875;0.01205156321038763043984598510860450915060937404632568359375;0.01278715178153389496473746334004317759536206722259521484375;0.01115871878165029806861952010876848362386226654052734375;-0.002859971099156568587196236563841011957265436649322509765625;-0.0019629482754365619630310124676952909794636070728302001953125;-0.0086151839933822187134193626434353063814342021942138671875;0.00174858440777187038213391634400295515661127865314483642578125;-0.01323180367395891676718377993893227539956569671630859375;0.00276938240801051678563471369898252305574715137481689453125;-0.00877533941830567661146478286582350847311317920684814453125;0.00268341621277570600845319148675116593949496746063232421875;0.0078330097519283721496652361793167074210941791534423828125;0.01056608133068198847326346623276549507863819599151611328125;0.00856310439247244363503153152805680292658507823944091796875;0.0037300890089778195903014168521849569515325129032135009765625;-0.0036564673780585909938778410577242539147846400737762451171875;0.00910931066802874063459416476007390883751213550567626953125;-0.004678353366452448793000318261192660429514944553375244140625;-0.0080094426535534286870632314503382076509296894073486328125;-0.0007558791140228862844019364075620615039952099323272705078125;0.006449121773167149594685465530119472532533109188079833984375;-0.00131600111876151756699904193936845331336371600627899169921875;0.00525732431395188604117407749072299338877201080322265625;0.001332551688508547445277674370345266652293503284454345703125;0.00427706480160073253260488712612641393207013607025146484375;-0.00950556679029437336103658395813909010030329227447509765625;0.005730426808411771821827329631560132838785648345947265625;0.00508392544602999894853834206287501729093492031097412109375;0.00506058440005886268908685821088511147536337375640869140625;0.011834339263637465300416096170010860078036785125732421875;-0.0003449992763752953383281363297641064491472207009792327880859375;-0.0114351107070735542869943657251496915705502033233642578125;0.00783101165138963377365666218565820599906146526336669921875;-0.01403100732721834949245920398652742733247578144073486328125;-0.004373402040658883570267700946487821056507527828216552734375;0.00822243007501474894305193430454892222769558429718017578125;-0.00102351186185454059475452570637798999086953699588775634765625;0.009431169907436365296149460846208967268466949462890625;0.0063451948741047557722705363403292722068727016448974609375;0.0041419120969572974233496864826520322822034358978271484375;-0.0035233659709833216149010848283751329290680587291717529296875;0.0116054220619492449995124871975349378772079944610595703125;-0.012943434681874775582510750382425612770020961761474609375;-0.01144783414304829764762683197432124870829284191131591796875;-0.0245514420394156891724879443472673301585018634796142578125;-0.005883344458003751664687541733655962161719799041748046875;0.00166971111128907793476339183058598791831173002719879150390625;0.0122237284889527286768640124137164093554019927978515625;0.01372193035965791653441048225658960291184484958648681640625;-0.006650703206520082282071637536091657239012420177459716796875;-0.00979041929095626935197760332130201277323067188262939453125;0.0018736226966915531071122824613439661334268748760223388671875;0.009417437572067553774868287064236938022077083587646484375;-0.01170226028499656012460405918318429030478000640869140625 ...(+2243 chars)]
      mask Display: e = 0.06;c1 = [120 150 230]/255;c2 = ([120 150 230]+0)/383;c3 = ([120 150 230]+128)/383;patch([0 1 1 0],[0 0 1 1],c1);patch([0 1 1 1-e 1-e 0+e],[0 0 1 1-e 0+e 0+e],c2);patch([0 0 1 1-e 0+e 0+e],[0 1 1 1-e 1-e 0+e],c3);plot([0 1 1 0 0],[0 0 1 1 0]);disp('b');
  netsum : Sum  Inputs=3  InputSameDT=on  SaturateOnIntegerOverflow=on  OutDataTypeStr=Inherit: Same as first input
      mask Display: e = 0.06;c1 = [120 150 230]/255;c2 = ([120 150 230]+0)/383;c3 = ([120 150 230]+128)/383;patch([0 1 1 0],[0 0 1 1],c1);patch([0 1 1 1-e 1-e 0+e],[0 0 1 1-e 0+e 0+e],c2);patch([0 0 1 1-e 0+e 0+e],[0 1 1 1-e 1-e 0+e],c3);plot([0 1 1 0 0],[0 0 1 1 0]);disp('+');
  tansig : neural/Transfer Functions/tansig
  "a{1}" : Outport  InitialOutput=[0;0;0;0;0;0;0;0;0;0;0;0;0;0;0;0;0;0;0;0;0;0;0;0;0;0;0;0;0;0;0;0;0;0;0;0;0;0;0;0;0;0;0;0;0;0;0;0;0;0;0;0;0;0;0;0;0;0;0;0;0;0;0;0;0;0;0;0;0;0;0;0;0;0;0;0;0;0;0;0;0;0;0;0;0;0;0;0;0;0;0;0;0;0;0;0;0;0;0;0]
      mask Display: e = 0.06;c1 = [120 230 180]/255;c2 = ([120 230 180]+0)/(256+128);c3 = ([120 230 180]+128)/(256+128);patch([0 1 1 0],[0 0 1 1],c1);patch([0 1 1 1-e 1-e 0+e],[0 0 1 1-e 0+e 0+e],c2);patch([0 0 1 1-e 0+e 0+e],[0 1 1 1-e 1-e 0+e],c3);plot([0 1 1 0 0],[0 0 1 1 0]);
  wires:
  tansig/1 -> "a{1}"/1
  netsum/1 -> tansig/1
  "b{1}"/1 -> netsum/3
  "IW{1,2}"/1("iz{1,2}") -> netsum/2
  Delays 2/1("pd{1,2}") -> "IW{1,2}"/1("pd{1,2}")
  "p{2}"/1 -> Delays 2/1("p{1}")
  "IW{1,1}"/1("iz{1,1}") -> netsum/1
  Delays 1/1("pd{1,1}") -> "IW{1,1}"/1("pd{1,1}")
  "p{1}"/1 -> Delays 1/1("p{1}")

== system MainSim/NARX Controller1/Layer 2 ==
  "a{1} " : Inport  PortDimensions=100  SampleTime=0.1
      mask Display: e = 0.06;c1 = [120 230 180]/255;c2 = ([120 230 180]+0)/(256+128);c3 = ([120 230 180]+128)/(256+128);patch([0 1 1 0],[0 0 1 1],c1);patch([0 1 1 1-e 1-e 0+e],[0 0 1 1-e 0+e 0+e],c2);patch([0 0 1 1-e 0+e 0+e],[0 1 1 1-e 1-e 0+e],c3);plot([0 1 1 0 0],[0 0 1 1 0]);
  Delays 1 : Subsystem
      mask Display: e = 0.06;c1 = [120 150 230]/255;c2 = ([120 150 230]+0)/383;c3 = ([120 150 230]+128)/383;patch([0 1 1 0],[0 0 1 1],c1);patch([0 1 1 1-e 1-e 0+e],[0 0 1 1-e 0+e 0+e],c2);patch([0 0 1 1-e 0+e 0+e],[0 1 1 1-e 1-e 0+e],c3);plot([0 1 1 0 0],[0 0 1 1 0]);disp('0');
  "LW{2,1}" : Subsystem
      mask Display: e = 0.06;c1 = [120 150 230]/255;c2 = ([120 150 230]+0)/383;c3 = ([120 150 230]+128)/383;patch([0 1 1 0],[0 0 1 1],c1);patch([0 1 1 1-e 1-e 0+e],[0 0 1 1-e 0+e 0+e],c2);patch([0 0 1 1-e 0+e 0+e],[0 1 1 1-e 1-e 0+e],c3);plot([0 1 1 0 0],[0 0 1 1 0]);disp('W');
  "b{2}" : Constant  Value=[-0.038746412276604295932269650393209303729236125946044921875;0.10887518811133491125620054162936867214739322662353515625;-0.04051718221217563697944541445394861511886119842529296875;-0.041253916418590740045058140594846918247640132904052734375;0.041980855311955021791359143890076666139066219329833984375]
      mask Display: e = 0.06;c1 = [120 150 230]/255;c2 = ([120 150 230]+0)/383;c3 = ([120 150 230]+128)/383;patch([0 1 1 0],[0 0 1 1],c1);patch([0 1 1 1-e 1-e 0+e],[0 0 1 1-e 0+e 0+e],c2);patch([0 0 1 1-e 0+e 0+e],[0 1 1 1-e 1-e 0+e],c3);plot([0 1 1 0 0],[0 0 1 1 0]);disp('b');
  netsum : Sum  Inputs=2  InputSameDT=on  SaturateOnIntegerOverflow=on  OutDataTypeStr=Inherit: Same as first input
      mask Display: e = 0.06;c1 = [120 150 230]/255;c2 = ([120 150 230]+0)/383;c3 = ([120 150 230]+128)/383;patch([0 1 1 0],[0 0 1 1],c1);patch([0 1 1 1-e 1-e 0+e],[0 0 1 1-e 0+e 0+e],c2);patch([0 0 1 1-e 0+e 0+e],[0 1 1 1-e 1-e 0+e],c3);plot([0 1 1 0 0],[0 0 1 1 0]);disp('+');
  purelin : neural/Transfer Functions/purelin
  "a{2}" : Outport  InitialOutput=[0;0;0;0;0]
      mask Display: e = 0.06;c1 = [120 230 180]/255;c2 = ([120 230 180]+0)/(256+128);c3 = ([120 230 180]+128)/(256+128);patch([0 1 1 0],[0 0 1 1],c1);patch([0 1 1 1-e 1-e 0+e],[0 0 1 1-e 0+e 0+e],c2);patch([0 0 1 1-e 0+e 0+e],[0 1 1 1-e 1-e 0+e],c3);plot([0 1 1 0 0],[0 0 1 1 0]);
  wires:
  purelin/1 -> "a{2}"/1
  netsum/1 -> purelin/1
  "b{2}"/1 -> netsum/2
  "LW{2,1}"/1("lz{2,1}") -> netsum/1
  Delays 1/1("pd{2,1}") -> "LW{2,1}"/1("ad{2,1}")
  "a{1} "/1 -> Delays 1/1("p{2}")

== system MainSim/NARX Controller1/Process Input 1 ==
  x : Inport  PortDimensions=12  SampleTime=0.1
      mask Display: e = 0.06;c1 = [120 230 180]/255;c2 = ([120 230 180]+0)/(256+128);c3 = ([120 230 180]+128)/(256+128);patch([0 1 1 0],[0 0 1 1],c1);patch([0 1 1 1-e 1-e 0+e],[0 0 1 1-e 0+e 0+e],c2);patch([0 0 1 1-e 0+e 0+e],[0 1 1 1-e 1-e 0+e],c3);plot([0 1 1 0 0],[0 0 1 1 0]);
  mapminmax : neural/Processing Functions/mapminmax  xmin=[-0.0129651907970248399248891502111;-0.169102256865743955094316675059;-0.000261394129407086525749420724551;-0.000200456542083920537114863358319;-0.0572538413172016327767899213086;-0.00259145694524988380244567842681;-0.00814332636769390071085350513158;-0.000996740230341396863528169447477;-0.0513394595556882285536381971269;-0.0447646016402733909478328655496;-0.052963182292912053261701998963;-0.0100089877342308310875784727045]  xmax=[0.0513394595556882285536381971269;0.00399453634531498312509878445553;6.63522293856221414068419228727e-05;0.00596627424954731047646028230247;0.0572499038085891240323910267307;0.00262231786722454379007229974263;0.000519043447362519381506340554466;0.0105862926184974084214962530837;0.0499577765287277028583012850049;0.177237932971395034664752188291;0.0529671449844292679953738911536;0.00997102928949204769804026682323]  ymin=-1  ymax=1
  p : Outport  PortDimensions=12  SampleTime=0.1
      mask Display: e = 0.06;c1 = [120 230 180]/255;c2 = ([120 230 180]+0)/(256+128);c3 = ([120 230 180]+128)/(256+128);patch([0 1 1 0],[0 0 1 1],c1);patch([0 1 1 1-e 1-e 0+e],[0 0 1 1-e 0+e 0+e],c2);patch([0 0 1 1-e 0+e 0+e],[0 1 1 1-e 1-e 0+e],c3);plot([0 1 1 0 0],[0 0 1 1 0]);
  wires:
  mapminmax/1 -> p/1
  x/1 -> mapminmax/1

== system MainSim/NARX Controller1/Process Input 2 ==
  x : Inport  PortDimensions=5  SampleTime=0.1
      mask Display: e = 0.06;c1 = [120 230 180]/255;c2 = ([120 230 180]+0)/(256+128);c3 = ([120 230 180]+128)/(256+128);patch([0 1 1 0],[0 0 1 1],c1);patch([0 1 1 1-e 1-e 0+e],[0 0 1 1-e 0+e 0+e],c2);patch([0 0 1 1-e 0+e 0+e],[0 1 1 1-e 1-e 0+e],c3);plot([0 1 1 0 0],[0 0 1 1 0]);
  mapminmax : neural/Processing Functions/mapminmax  xmin=[-0.20244393015821871006920673608;-0.000162983708575139977017820491767;-0.493690097282159567892989571192;-0.2162391512775998225759366278;-0.00605850883196610689312988640154]  xmax=[0.00478930326934306517527861757344;0.00152521114561354753647037796327;0.0115063547556192961873744451395;0.00507127823624882630160204399772;0.226011889004929134028287762703]  ymin=-1  ymax=1
  p : Outport  PortDimensions=5  SampleTime=0.1
      mask Display: e = 0.06;c1 = [120 230 180]/255;c2 = ([120 230 180]+0)/(256+128);c3 = ([120 230 180]+128)/(256+128);patch([0 1 1 0],[0 0 1 1],c1);patch([0 1 1 1-e 1-e 0+e],[0 0 1 1-e 0+e 0+e],c2);patch([0 0 1 1-e 0+e 0+e],[0 1 1 1-e 1-e 0+e],c3);plot([0 1 1 0 0],[0 0 1 1 0]);
  wires:
  mapminmax/1 -> p/1
  x/1 -> mapminmax/1

== system MainSim/NARX Controller1/Process Output 1 ==
  a : Inport  PortDimensions=5  SampleTime=0.1
      mask Display: e = 0.06;c1 = [120 230 180]/255;c2 = ([120 230 180]+0)/(256+128);c3 = ([120 230 180]+128)/(256+128);patch([0 1 1 0],[0 0 1 1],c1);patch([0 1 1 1-e 1-e 0+e],[0 0 1 1-e 0+e 0+e],c2);patch([0 0 1 1-e 0+e 0+e],[0 1 1 1-e 1-e 0+e],c3);plot([0 1 1 0 0],[0 0 1 1 0]);
  mapminmax_reverse : neural/Processing Functions/mapminmax_reverse  xmin=[-0.20244393015821871006920673608;-0.000162983708575139977017820491767;-0.493690097282159567892989571192;-0.2162391512775998225759366278;-0.00605850883196610689312988640154]  xmax=[0.00478930326934306517527861757344;0.00152521114561354753647037796327;0.0115063547556192961873744451395;0.00507127823624882630160204399772;0.226011889004929134028287762703]  ymin=-1  ymax=1
  y : Outport  PortDimensions=5  SampleTime=0.1
      mask Display: e = 0.06;c1 = [120 230 180]/255;c2 = ([120 230 180]+0)/(256+128);c3 = ([120 230 180]+128)/(256+128);patch([0 1 1 0],[0 0 1 1],c1);patch([0 1 1 1-e 1-e 0+e],[0 0 1 1-e 0+e 0+e],c2);patch([0 0 1 1-e 0+e 0+e],[0 1 1 1-e 1-e 0+e],c3);plot([0 1 1 0 0],[0 0 1 1 0]);
  wires:
  mapminmax_reverse/1 -> y/1
  a/1 -> mapminmax_reverse/1
